simulink model "Application"  (R2018a)
settings: Solver=ode8  StartTime=0.0  StopTime=Ttot  FixedStep=Ts  RelTol=1e-3  AbsTol=2e-5
values from neighbouring files (symbols this model uses):
  Cdc = 1 / (2 * pi * Fn * 5)    (= 0.000530516476973)    [Application_Script.m]
  DualType = 2    [Application_Script.m]
  Fdroop = 1e10    (= 10000000000)    [Application_Script.m]
  Fdrop = -0.01    [Application_Script.m]
  Fdroptime = 0.75    [Application_Script.m]
  FixedDC = 0    [Application_Script.m]
  Fn = 60    [Application_Script.m]    (also in ShortPulse_Script.m)
  Frampslope = -Fdrop / 2    (= 0.005)    [Application_Script.m]
  Idc = 1.5/Udc    (= 0.866025403784)    [Application_Script.m]
  Kpdc = 0.5    [Application_Script.m]
  L = X / 2 / pi / Fn    (= 0.00132629119243)    [Application_Script.m]
  PdcFinVal = 0.0    (= 0)    [Application_Script.m]
  PdcIniVal = 0    [Application_Script.m]
  PdcStepTime = 0.00    (= 0)    [Application_Script.m]
  R = X / 20    (= 0.025)    [Application_Script.m]
  Ts = Ts_control / 60    (= 9.25925925926e-07)    [Application_Script.m]    (also in ShortPulse_Script.m)
  Ts_control = 1/(300*Fn)    (= 5.55555555556e-05)    [Application_Script.m]    (also in ShortPulse_Script.m)
  Udc = 3^0.5    (= 1.73205080757)    [Application_Script.m]
  VarDC = 1    [Application_Script.m]
undefined symbols (not defined in the file or in its folder): ESS, PCC
libraries: powerlib x15, DSCdq_Library x6, powerlib_meascontrol x5, simulink x1
settings Model: SimulationMode=accelerator  Creator=daniemot  LastModifiedBy=daniemot
settings SolverCC: AutoInsertRateTranBlk=on
settings DataIOCC: ExternalInput=getinputstruct(WN_50mF_op_snapshot1)  InitialState=getstatestruct(WN_50mF_op_snapshot1)  SaveFinalState=on  SaveFormat=StructureWithTime  SaveOutput=off  SignalLogging=off  DSMLogging=off  SaveTime=off
settings DebuggingCC: ReadBeforeWriteMsg=DisableAll  WriteAfterWriteMsg=DisableAll  WriteAfterReadMsg=DisableAll  MultiTaskDSMMsg=none  UnconnectedInputMsg=none  UnconnectedOutputMsg=none  UnconnectedLineMsg=none
settings ModelReferenceCC: UpdateModelReferenceTargets=IfOutOfDate
settings SFSimCC: SFSimEcho=off

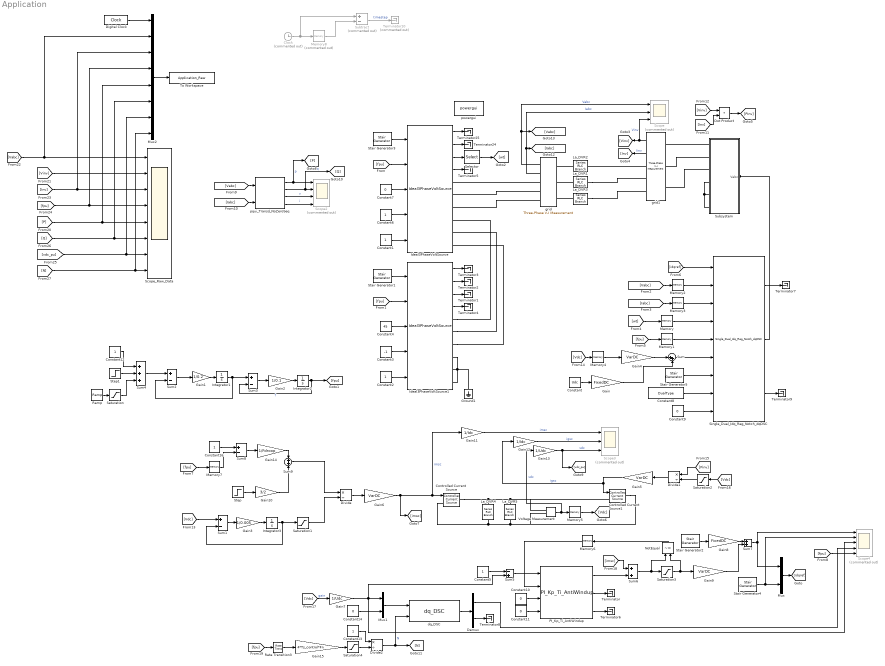
== system Application ==
  Clock : Clock  Commented=on
  Constant : Constant  Value=Udc
  Constant{1..2,5..6,12..13,16} (7 alike) : Constant
  Constant{7,9..11,14} (5 alike) : Constant  Value=0
  Constant3 : Constant  Value=-1
  Constant4 : Constant  Value=45
  Constant8 : Constant  Value=DualType
  Controlled Current Source : powerlib/Electrical Sources/Controlled Current Source  Initialize=on  Source_Type=AC  Amplitude=0  Phase=0  Frequency=0  Measurements=None
  Controlled Current Source1 : powerlib/Electrical Sources/Controlled Current Source  Initialize=on  Source_Type=AC  Amplitude=0  Phase=0  Frequency=0  Measurements=None
  Demux : Demux  Outputs=2
  Digital Clock : DigitalClock  SampleTime=Ts_control
  Divide : Product  Inputs=*/
  Divide1 : Product  Inputs=*/
  Divide2 : Product  Inputs=*/
  Dot Product : DotProduct  InputSameDT=on  OutDataTypeStr=Inherit: Inherit via internal rule
  Gain : Gain  Gain=FixedDC
  Gain1 : Gain  Gain=1/0.2
  Gain10 : Gain  Gain=3/2
  Gain11 : Gain  Gain=1/Idc
  Gain12 : Gain  Gain=1/Idc
  Gain13 : Gain  Gain=1/Udc
  Gain14 : Gain  Gain=1/Fdroop
  Gain15 : Gain  Gain=4*Ts_control*Fn
  Gain2 : Gain  Gain=1/0.1
  Gain3 : Gain  Gain=1/0.005
  Gain{4..6,9} (4 alike) : Gain  Gain=VarDC
  Gain7 : Gain  Gain=1/Udc
  Gain8 : Gain  Gain=FixedDC
  Ground1 : powerlib/Elements/Ground  LConnTagsString=a
  Ideal3PhaseVoltSource : DSCdq_Library/Ideal3PhaseVoltSource  BaseAmp=1  fn=Fn
  Ideal3PhaseVoltSource1 : DSCdq_Library/Ideal3PhaseVoltSource  BaseAmp=1  fn=Fn
  Integrator1 : Integrator  InitialCondition=1
  Integrator2 : Integrator  InitialCondition=1
  Integrator3 : Integrator  InitialCondition=Udc
  La_DVR1 : powerlib/Elements/Series RLC Branch  LConnTagsString=__new0  RConnTagsString=__new0  BranchType=RL  Resistance=R  Inductance=L  SetiL0=off  InitialCurrent=0  Capacitance=1.0  Setx0=off  InitialVoltage=0  Measurements=None
  La_DVR2 : powerlib/Elements/Series RLC Branch  LConnTagsString=__new0  RConnTagsString=__new0  BranchType=RL  Resistance=R  Inductance=L  SetiL0=off  InitialCurrent=0  Capacitance=1.0  Setx0=off  InitialVoltage=0  Measurements=None
  La_DVR3 : powerlib/Elements/Series RLC Branch  LConnTagsString=__new0  RConnTagsString=__new0  BranchType=RL  Resistance=R  Inductance=L  SetiL0=off  InitialCurrent=0  Capacitance=1.0  Setx0=off  InitialVoltage=0  Measurements=None
  La_DVR4 : powerlib/Elements/Series RLC Branch  LConnTagsString=__new0  RConnTagsString=__new0  BranchType=C  Resistance=R  Inductance=L  SetiL0=off  InitialCurrent=0  Capacitance=Cdc  Setx0=on  InitialVoltage=Udc  Measurements=None
  La_DVR5 : powerlib/Elements/Series RLC Branch  LConnTagsString=__new0  RConnTagsString=__new0  BranchType=R  Resistance=1e6  Inductance=L  SetiL0=off  InitialCurrent=0  Capacitance=1  Setx0=on  InitialVoltage=1  Measurements=None
  Memory{,2..4,6} (5 alike) : Memory
  Memory1 : Memory  InitialCondition=1
  Memory5 : Memory  InitialCondition=1
  Memory7 : Memory  InitialCondition=1
  Memory8 : Memory  Commented=on
  Mux : Mux  Inputs=2
  Mux1 : Mux  Inputs=2
  Mux2 : Mux  Inputs=8
  NotEqual : RelationalOperator  Operator=~=  OutDataTypeStr=boolean  RndMeth=Simplest
  PI_Kp_Ti_AntiWindup : DSCdq_Library/PI_Kp_Ti_AntiWindup  Ts=Ts_control  Kp=Kpdc  Ti=Tidc  PI_max=1.5  PI_min=-1.5
  Ramp : simulink/Sources/Ramp  slope=Frampslope  start=Framptime  InitialOutput=0
  Rate Transition3 : RateTransition  InitialCondition=1  OutPortSampleTime=Ts_control
  Saturation : Saturate  UpperLimit=abs(Fdrop)  LowerLimit=-abs(Fdrop)
  Saturation1 : Saturate  UpperLimit=Inf  LowerLimit=1e-6
  Saturation2 : Saturate  UpperLimit=Inf  LowerLimit=1e-6
  Saturation3 : Saturate  UpperLimit=1.5  LowerLimit=-1.5
  Saturation4 : Saturate  UpperLimit=inf  LowerLimit=0.000001
  Scope : Scope  Commented=on  NumInputPorts=3
  Scope2 : Scope  Commented=on  NumInputPorts=4
  Scope3 : Scope  Commented=on  NumInputPorts=3
  Scope4 : Scope  Commented=on  NumInputPorts=5
  Scope_Raw_Data : Scope  NumInputPorts=8
  Selector : Selector  InputPortWidth=3  IndexOptions=Index vector (dialog)  Indices=[1]  OutputSizes=1
  Single_Dual_Idq_Reg_Notch_dqDSC : DSCdq_Library/Single_Dual_Idq_Reg_Notch_dqDSC  Ts=Ts_control  fgrid=Fn  fmin=Fmin  zetanotch=zeta  fcutout=Fcutout  PI_Kp=Kp  PI_Ti=Ti  PI_X=X  PI_max=1.5  PI_min=-1.5  PWM_Ts=Ts  PWM_fsw=Fsw  PWM_Uabp=3^0.5  PWM_Ini=90
  Stair Generator1 : powerlib_meascontrol/Pulse & Signal Generators/Stair Generator  t=VnegStepTimes  e=VnegStepValues  Ts=0
      settings: SourceProductName=Simscape Power Systems
  Stair Generator2 : powerlib_meascontrol/Pulse & Signal Generators/Stair Generator  t=IdStepTimes  e=IdStepValues  Ts=0
      settings: SourceProductName=Simscape Power Systems
  Stair Generator3 : powerlib_meascontrol/Pulse & Signal Generators/Stair Generator  t=VposStepTimes  e=VposStepValues  Ts=0
      settings: SourceProductName=Simscape Power Systems
  Stair Generator4 : powerlib_meascontrol/Pulse & Signal Generators/Stair Generator  t=IqStepTimes  e=IqStepValues  Ts=0
      settings: SourceProductName=Simscape Power Systems
  Stair Generator5 : powerlib_meascontrol/Pulse & Signal Generators/Stair Generator  t=EnDualTimes  e=EnDualValues  Ts=0
      settings: SourceProductName=Simscape Power Systems
  Step : Step  Time=PdcStepTime  Before=PdcIniVal  After=PdcFinVal  SampleTime=0
  Step1 : Step  Time=Fdroptime  After=-Fdrop  SampleTime=0
  Subsystem : Subsystem
  Subtract : Sum  Commented=on  Inputs=+-
  Sum : Sum  Inputs=|++
  Sum{1..3,8} (4 alike) : Sum  Inputs=+-
  Sum4 : Sum  Inputs=+++
  Sum5 : Sum  Inputs=-+
  Sum6 : Sum
  Sum7 : Sum
  Sum9 : Sum
  Terminator{,1..9,24..25} (12 alike) : Terminator
  Terminator10 : Terminator  Commented=on
  To Workspace : ToWorkspace  VariableName=Application_Raw  SampleTime=Ts_control
  Voltage Measurement : powerlib/Measurements/Voltage Measurement  PhasorSimulation=off  OutputType=Complex  PSBequivalent=0
  dq_DSC : DSCdq_Library/dq_DSC  Ts=Ts_control  nmax=400
  grid : powerlib/Measurements/Three-Phase V-I Measurement  VoltageMeasurement=phase-to-ground  SetLabelV=off  LabelV=vgrid  Vpu=off  VpuLL=off  CurrentMeasurement=yes  SetLabelI=off  LabelI=igrid  Ipu=off  Pbase=sn  Vbase=uab  OutputType=Complex  PhasorSimulation=off  PSBequivalent=0
  grid1 : powerlib/Measurements/Three-Phase V-I Measurement  VoltageMeasurement=phase-to-ground  SetLabelV=off  LabelV=vconv  Vpu=off  VpuLL=off  CurrentMeasurement=yes  SetLabelI=off  LabelI=iconv  Ipu=off  Pbase=sn  Vbase=uab  OutputType=Complex  PhasorSimulation=off  PSBequivalent=0
  powergui : powerlib/powergui  Priority=1  SimulationMode=Discrete  SampleTime=Ts  frequency=60  Iterations=50  frequencyindice=0  Pbase=100e6  ErrMax=1e-4  UnitsV=kV  UnitsW=MW  buscounter=0  FunctionMessages=off  echomessages=off  EnableUseOfTLC=off  CurrentSourceSwitches=off  DisableSnubberDevices=off  DisableRonSwitches=off  DisableVfSwitches=off  DisplayEquations=off  SolverType=Tustin/Backward Euler (TBE)  Interpol=off  ExternalGateDelay=off  methode=off  Ts=100  x0status=blocks  SPID=off  SwTol=0  HookPort=off  RestoreLinks=warning  ResistiveCurrentMeasurement=off  Frange=[60:1:1600]  Ylog=on  Xlog=on  ShowGrid=on  save=off  variable=ZData  structure=0  ZoomFFT=off  StartTime=0.0  cycles=1  DisplayStyle=1  fundamental=60  FreqAxis=off  MaxFrequency=1000  frequencyindicesteady=1  RmsSteady=1  display=off
  pqui_Transd_NoZeroSeq : DSCdq_Library/pqui_Transd_NoZeroSeq  Sn=3/2  Uanp=1  Iap=1
  wires:
  Constant6/1 -> Ideal3PhaseVoltSource/4
  Constant7/1 -> Ideal3PhaseVoltSource/3
  [fpu] -> Ideal3PhaseVoltSource/2
  Ideal3PhaseVoltSource/3 -> Selector/1
  Ideal3PhaseVoltSource/2 -> Terminator24/1
  Ideal3PhaseVoltSource/1 -> Terminator25/1
  Ideal3PhaseVoltSource/4 -> Terminator5/1
  Stair Generator3/1 -> Ideal3PhaseVoltSource/1
  Constant1/1 -> Ideal3PhaseVoltSource/5
  Integrator2/1 -> Sum3/2, [fpu]  "f"
  Integrator1/1 -> Sum2/2, Sum3/1
  Step1/1 -> Sum4/2
  Gain2/1 -> Integrator2/1
  Sum2/1 -> Gain1/1
  Sum4/1 -> Sum2/1
  Constant12/1 -> Sum4/1
  Ramp/1 -> Saturation/1
  Saturation/1 -> Sum4/3
  Sum3/1 -> Gain2/1
  Gain1/1 -> Integrator1/1
  [fpu] -> Ideal3PhaseVoltSource1/2
  Constant4/1 -> Ideal3PhaseVoltSource1/3
  Ideal3PhaseVoltSource1/2 -> Terminator2/1
  Constant3/1 -> Ideal3PhaseVoltSource1/4
  Ideal3PhaseVoltSource1/1 -> Terminator3/1
  Constant2/1 -> Ideal3PhaseVoltSource1/5
  Stair Generator1/1 -> Ideal3PhaseVoltSource1/1
  Ideal3PhaseVoltSource1/4 -> Terminator4/1
  Ideal3PhaseVoltSource1/3 -> Terminator1/1
  grid/2 -> Scope/2, [Iabc]  "Iabc"
  grid/1 -> Scope/1, [Vabc]  "Vabc"
  grid1/1 -> [Vinv], Scope/3  "Vinv"
  grid1/2 -> [Inv]  "Iinv"
  Stair Generator2/1 -> Gain8/1
  Stair Generator4/1 -> Scope4/2, Mux/2
  Mux/1 -> [idqref]
  [Vabc] -> Memory2/1
  [Iabc] -> Memory3/1
  Selector/1 -> [wt]
  [wt] -> Memory/1
  [fpu] -> Memory1/1
  Sum/1 -> Single_Dual_Idq_Reg_Notch_dqDSC/6
  Stair Generator5/1 -> Single_Dual_Idq_Reg_Notch_dqDSC/7
  Constant8/1 -> Single_Dual_Idq_Reg_Notch_dqDSC/8
  Constant9/1 -> Single_Dual_Idq_Reg_Notch_dqDSC/9
  [idqref] -> Single_Dual_Idq_Reg_Notch_dqDSC/1
  Single_Dual_Idq_Reg_Notch_dqDSC/3 -> Terminator9/1
  Single_Dual_Idq_Reg_Notch_dqDSC/2 -> Subsystem/1(Vabc)
  Single_Dual_Idq_Reg_Notch_dqDSC/1 -> Terminator7/1
  Memory/1 -> Single_Dual_Idq_Reg_Notch_dqDSC/4
  Memory1/1 -> Single_Dual_Idq_Reg_Notch_dqDSC/5
  Memory2/1 -> Single_Dual_Idq_Reg_Notch_dqDSC/2
  Memory3/1 -> Single_Dual_Idq_Reg_Notch_dqDSC/3
  [fpu] -> Scope4/5
  [Vabc] -> pqui_Transd_NoZeroSeq/1
  [Iabc] -> pqui_Transd_NoZeroSeq/2
  pqui_Transd_NoZeroSeq/1 -> [P], Scope2/1  "p"
  pqui_Transd_NoZeroSeq/2 -> [Q], Scope2/2  "q"
  pqui_Transd_NoZeroSeq/3 -> Scope2/3  "v"
  pqui_Transd_NoZeroSeq/4 -> Scope2/4  "i"
  [Vinv] -> Dot Product/1
  [Inv] -> Dot Product/2
  Dot Product/1 -> [Pinv]
  Voltage Measurement/1 -> Gain13/1, Memory5/1  "vdc"
  Sum1/1 -> Gain3/1
  Integrator3/1 -> Saturation1/1, Sum1/2
  Gain3/1 -> Integrator3/1
  Divide/1 -> Gain6/1
  [Vdc] -> Memory4/1
  Constant/1 -> Gain/1
  Memory4/1 -> Gain4/1
  Gain4/1 -> Sum/1
  Gain/1 -> Sum/2
  Divide1/1 -> Gain5/1
  [Pinv] -> Divide1/1
  Saturation2/1 -> Divide1/2
  Gain5/1 -> Gain12/1, Controlled Current Source1/1  "igsc"
  Gain6/1 -> [imsc], Gain11/1, Controlled Current Source/1  "imsc"
  Memory5/1 -> [Vdc]
  [Vdc] -> Gain7/1  "gain"
  Constant5/1 -> Sum5/1
  Sum5/1 -> PI_Kp_Ti_AntiWindup/1
  Constant10/1 -> PI_Kp_Ti_AntiWindup/3
  Constant11/1 -> PI_Kp_Ti_AntiWindup/4
  PI_Kp_Ti_AntiWindup/1 -> Sum6/2
  [imsc] -> Sum6/1
  PI_Kp_Ti_AntiWindup/2 -> Terminator/1
  PI_Kp_Ti_AntiWindup/3 -> Terminator6/1
  Sum6/1 -> NotEqual/1, Saturation3/1
  Saturation3/1 -> Gain9/1, NotEqual/2
  NotEqual/1 -> Memory6/1
  Gain8/1 -> Sum7/1
  Gain9/1 -> Sum7/2
  Sum7/1 -> Scope4/1, Mux/1
  Memory6/1 -> PI_Kp_Ti_AntiWindup/2
  Step/1 -> Gain10/1
  [Vdc] -> Sum1/1
  Gain11/1 -> Scope3/1  "imsc"
  Gain12/1 -> Scope3/2  "igsc"
  Gain13/1 -> [vdc_pu], Scope3/3  "vdc"
  Gain10/1 -> Sum9/2
  Gain15/1 -> Saturation4/1
  Saturation4/1 -> Divide2/2
  Rate Transition3/1 -> Gain15/1
  Constant13/1 -> Divide2/1
  [fpu] -> Rate Transition3/1
  Divide2/1 -> [N], dq_DSC/2  "N"
  Mux1/1 -> dq_DSC/1
  Constant14/1 -> Mux1/2
  Gain7/1 -> Sum5/2, Mux1/1, Scope4/3
  dq_DSC/1 -> Demux/1
  Demux/2 -> Terminator8/1
  Demux/1 -> Scope4/4
  Saturation1/1 -> Divide/2
  Constant16/1 -> Sum8/1
  [fpu] -> Memory7/1
  Memory7/1 -> Sum8/2
  Sum8/1 -> Gain14/1
  Gain14/1 -> Sum9/1
  Sum9/1 -> Divide/1
  [Vabc] -> Mux2/2, Scope_Raw_Data/1
  [Vinv] -> Scope_Raw_Data/2
  [Inv] -> Mux2/3, Scope_Raw_Data/3
  [fpu] -> Mux2/4, Scope_Raw_Data/4
  [P] -> Mux2/5, Scope_Raw_Data/5
  [vdc_pu] -> Mux2/7, Scope_Raw_Data/7
  [Q] -> Mux2/6, Scope_Raw_Data/6
  [N] -> Mux2/8, Scope_Raw_Data/8
  Mux2/1 -> To Workspace/1
  Digital Clock/1 -> Mux2/1
  [Vdc] -> Saturation2/1
  Clock/1 -> Subtract/1, Memory8/1
  Memory8/1 -> Subtract/2
  Subtract/1 -> Terminator10/1  "timestep"
  connections:
  Ideal3PhaseVoltSource1/RConn2 -- Ideal3PhaseVoltSource/RConn5
  Ideal3PhaseVoltSource1/RConn1 -- Ideal3PhaseVoltSource/RConn4
  Ideal3PhaseVoltSource1/RConn3 -- Ideal3PhaseVoltSource/RConn6
  Ideal3PhaseVoltSource1/RConn4 -- Ground1/LConn1 -- Ideal3PhaseVoltSource1/RConn6 -- Ideal3PhaseVoltSource1/RConn5
  grid/RConn1 -- Ideal3PhaseVoltSource/RConn1
  grid/RConn2 -- Ideal3PhaseVoltSource/RConn2
  grid/RConn3 -- Ideal3PhaseVoltSource/RConn3
  La_DVR2/RConn1 -- grid/LConn1
  La_DVR3/RConn1 -- grid/LConn3
  La_DVR1/RConn1 -- grid/LConn2
  Subsystem/RConn5 -- Subsystem/RConn4 -- Subsystem/RConn6
  Subsystem/RConn1 -- grid1/LConn1
  Subsystem/RConn2 -- grid1/LConn2
  Subsystem/RConn3 -- grid1/LConn3
  grid1/RConn1 -- La_DVR2/LConn1
  La_DVR1/LConn1 -- grid1/RConn2
  La_DVR3/LConn1 -- grid1/RConn3
  La_DVR4/LConn1 -- Controlled Current Source/RConn1 -- Controlled Current Source1/LConn1 -- Voltage Measurement/LConn1 -- La_DVR5/LConn1
  La_DVR5/RConn1 -- Controlled Current Source1/RConn1 -- Voltage Measurement/LConn2 -- Controlled Current Source/LConn1 -- La_DVR4/RConn1

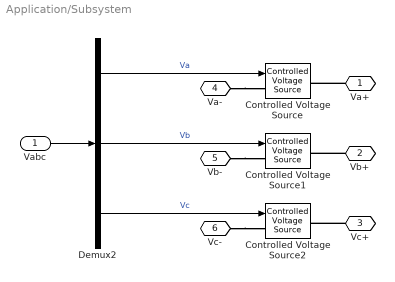
== system Application/Subsystem ==
  Vabc : Inport
  Controlled Voltage Source : powerlib/Electrical Sources/Controlled Voltage Source  Initialize=off  Source_Type=AC  Amplitude=ESS.LSC.Ub*(2/3)^0.5  Phase=0  Frequency=PCC.fn  Measurements=None
  Controlled Voltage Source1 : powerlib/Electrical Sources/Controlled Voltage Source  Initialize=off  Source_Type=AC  Amplitude=ESS.LSC.Ub*(2/3)^0.5  Phase=-120  Frequency=PCC.fn  Measurements=None
  Controlled Voltage Source2 : powerlib/Electrical Sources/Controlled Voltage Source  Initialize=off  Source_Type=AC  Amplitude=ESS.LSC.Ub*(2/3)^0.5  Phase=120  Frequency=PCC.fn  Measurements=None
  Demux2 : Demux  Outputs=3
  Va+ : PMIOPort  Side=Right
  Vb+ : PMIOPort  Port=2  Side=Right
  Vc+ : PMIOPort  Port=3  Side=Right
  Va- : PMIOPort  Port=4  Side=Right
  Vb- : PMIOPort  Port=5  Side=Right
  Vc- : PMIOPort  Port=6  Side=Right
  wires:
  Demux2/1 -> Controlled Voltage Source/1  "Va"
  Demux2/2 -> Controlled Voltage Source1/1  "Vb"
  Demux2/3 -> Controlled Voltage Source2/1  "Vc"
  Vabc/1 -> Demux2/1
  connections:
  Va-/RConn1 -- Controlled Voltage Source/LConn1
  Va+/RConn1 -- Controlled Voltage Source/RConn1
  Vb-/RConn1 -- Controlled Voltage Source1/LConn1
  Vc-/RConn1 -- Controlled Voltage Source2/LConn1
  Vb+/RConn1 -- Controlled Voltage Source1/RConn1
  Vc+/RConn1 -- Controlled Voltage Source2/RConn1
